simulink model "Project1_Part2_Op3"  (R2023b)
settings: Solver=ode45  StartTime=0.0  StopTime=25  FixedStep=1  RelTol=1e-3
values from neighbouring files (symbols this model uses):
  b1 = 1    [Project1_Part2.m]
  b2 = 1    [Project1_Part2.m]
  const_torque = 1    [Project1_Part2.m]
  J1 = 100    [Project1_Part2.m]
  J2 = 1    [Project1_Part2.m]
  omega0 = 0    [Project1_Part2.m]
  theta0 = 0    [Project1_Part2.m]
settings Model: Creator=flare  LastModifiedBy=flare

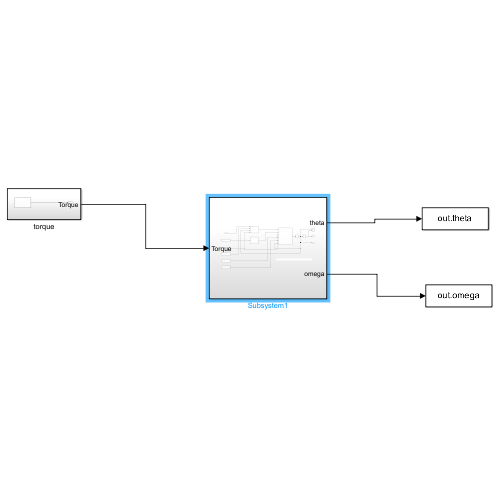
[thumbnail: Simulink's stored preview of the top-level diagram]
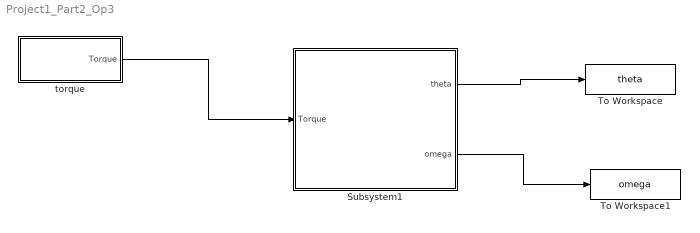
== system Project1_Part2_Op3 ==
  Subsystem1 : Subsystem
  To Workspace : ToWorkspace  VariableName=theta  SaveFormat=Timeseries  SampleTime=-1
  To Workspace1 : ToWorkspace  VariableName=omega  SaveFormat=Timeseries  SampleTime=-1
  torque : Subsystem
  wires:
  torque/1(Torque) -> Subsystem1/1(Torque)
  Subsystem1/1(theta) -> To Workspace/1
  Subsystem1/2(omega) -> To Workspace1/1

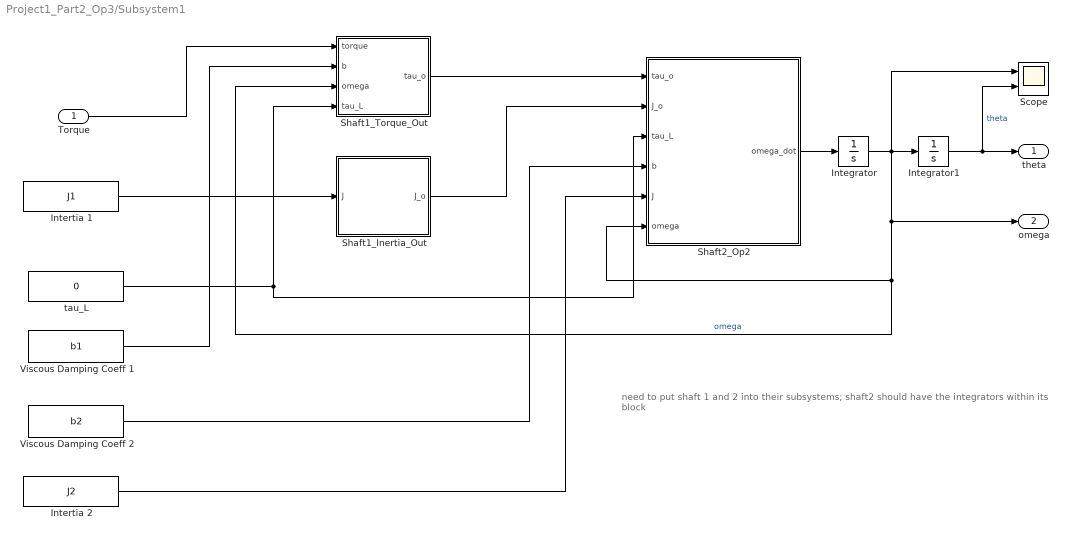
== system Project1_Part2_Op3/Subsystem1 ==
  note: need to put shaft 1 and 2 into their subsystems; shaft2 should have the integrators within its block
  Torque : Inport
  Integrator : Integrator  InitialCondition=omega0
  Integrator1 : Integrator  InitialCondition=theta0
  Intertia 1 : Constant  Value=J1
  Intertia 2 : Constant  Value=J2
  Scope : Scope  NumInputPorts=2
  Shaft1_Inertia_Out : MATLAB Function  TreatAsAtomicUnit=on
  Shaft1_Torque_Out : MATLAB Function  TreatAsAtomicUnit=on
  Shaft2_Op2 : MATLAB Function  TreatAsAtomicUnit=on
  Viscous Damping Coeff 1 : Constant  Value=b1
  Viscous Damping Coeff 2 : Constant  Value=b2
  tau_L : Constant  Value=0
  theta : Outport
  omega : Outport  Port=2
  wires:
  Viscous Damping Coeff 1/1 -> Shaft1_Torque_Out/2(b)
  Integrator/1 -> Scope/1, omega/1, Shaft1_Torque_Out/3(omega), Shaft2_Op2/6(omega), Integrator1/1  "omega"
  Shaft2_Op2/1(omega_dot) -> Integrator/1
  Torque/1 -> Shaft1_Torque_Out/1(torque)
  tau_L/1 -> Shaft2_Op2/3(tau_L), Shaft1_Torque_Out/4(tau_L)
  Shaft1_Torque_Out/1(tau_o) -> Shaft2_Op2/1(tau_o)
  Shaft1_Inertia_Out/1(J_o) -> Shaft2_Op2/2(J_o)
  Intertia 1/1 -> Shaft1_Inertia_Out/1(J)
  Integrator1/1 -> Scope/2, theta/1  "theta"
  Viscous Damping Coeff 2/1 -> Shaft2_Op2/4(b)
  Intertia 2/1 -> Shaft2_Op2/5(J)

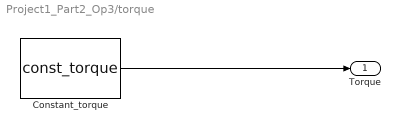
== system Project1_Part2_Op3/torque ==
  Constant_torque : Constant  Value=const_torque
  Torque : Outport
  wires:
  Constant_torque/1 -> Torque/1

== matlab function Project1_Part2_Op3/Subsystem1/Shaft2_Op2 ==
  data: tau_o input; J_o input; omega_dot output; tau_L input; b input; J input; omega input
function omega_dot = fcn(tau_o, J_o, tau_L, b, J, omega)

omega_dot = (tau_o + tau_L - b*omega)/(J + J_o);

== matlab function Project1_Part2_Op3/Subsystem1/Shaft1_Torque_Out ==
  data: torque input; tau_o output; b input; omega input; tau_L input
function tau_o = fcn(torque, b, omega, tau_L)

tau_o = torque - b*omega - tau_L;

== matlab function Project1_Part2_Op3/Subsystem1/Shaft1_Inertia_Out ==
  data: J input; J_o output
function J_o = fcn(J)

J_o = J;
